simulink model "SimulinkSerial"  (R2019a)
settings: Solver=VariableStepAuto  StartTime=0.0  StopTime=inf  RelTol=1e-3
undefined symbols (not defined in the file): serial
libraries: instrumentlib x2
settings Model: Creator=JackyL  LastModifiedBy=Administrator
settings DataIOCC: ReturnWorkspaceOutputs=off
settings DebuggingCC: ArithmeticOperatorsInVariantConditions=warning

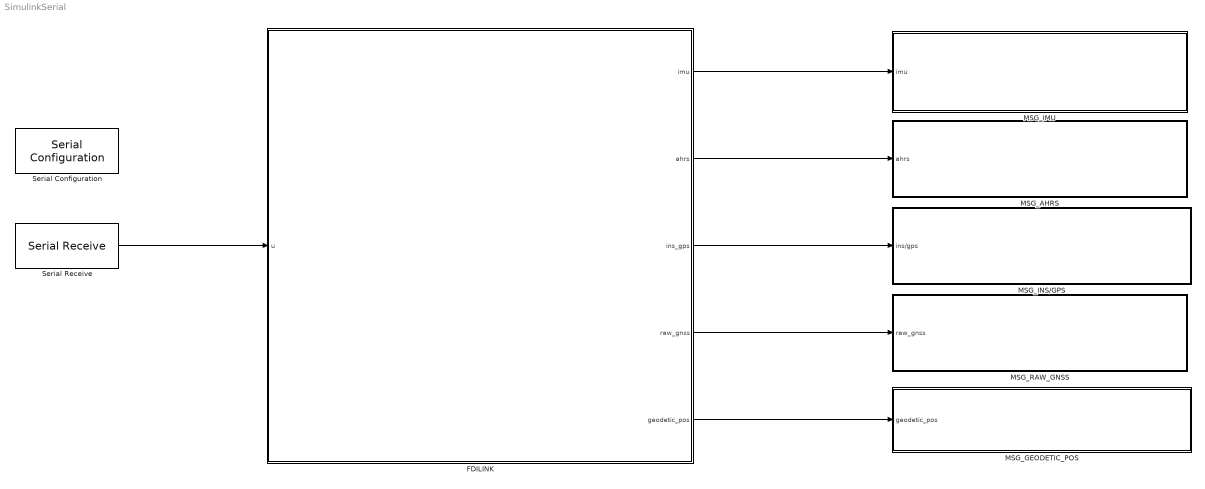
== system SimulinkSerial ==
  FDILINK : MATLAB Function  TreatAsAtomicUnit=on
  "MSG_AHRS " : Subsystem
  MSG_GEODETIC_POS : Subsystem
  "MSG_IMU " : Subsystem
  MSG_INS/GPS : Subsystem
  MSG_RAW_GNSS : Subsystem
  Serial Configuration : instrumentlib/Serial Configuration  Priority=-200000  ComPortMenu=<Please select a port...>  ComPort=COM2  ObjConstructor=serial('COM2');  BaudRate=921600  DataBits=8  Parity=none  StopBits=1  FlowControl=none  Timeout=10  ByteOrder=LittleEndian
  Serial Receive : instrumentlib/Serial Receive  ComPortMenu=COM2  ComPort=COM2  ObjConstructor=serial('COM2');  Terminator=<none>  DataSize="[1  200]"  DataType=uint8  EnableBlockingMode=on  ActionDataUnavailable=Output last received value  CustomValue=0  SampleTime=1
  wires:
  Serial Receive/1 -> FDILINK/1(u)
  FDILINK/1(imu) -> "MSG_IMU "/1("imu ")
  FDILINK/2(ahrs) -> "MSG_AHRS "/1("ahrs ")
  FDILINK/3(ins_gps) -> MSG_INS/GPS/1("ins/gps ")
  FDILINK/5(geodetic_pos) -> MSG_GEODETIC_POS/1("geodetic_pos ")
  FDILINK/4(raw_gnss) -> MSG_RAW_GNSS/1("raw_gnss ")

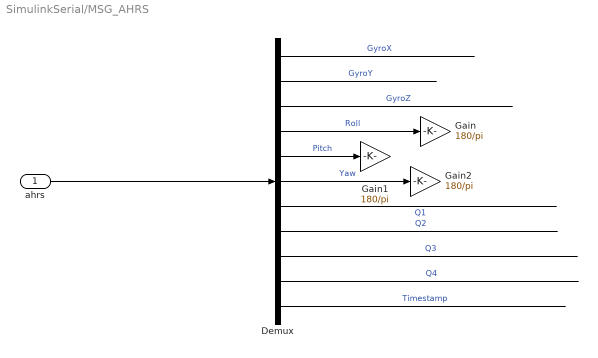
== system SimulinkSerial/MSG_AHRS  ==
  "ahrs " : Inport
  Demux : Demux  Outputs=11
  Gain : Gain  Gain=180/pi
  Gain1 : Gain  Gain=180/pi
  Gain2 : Gain  Gain=180/pi
  wires:
  "ahrs "/1 -> Demux/1
  Demux/1 -> ?  "GyroX"
  Demux/2 -> ?  "GyroY"
  Demux/3 -> ?  "GyroZ"
  Demux/5 -> Gain1/1  "Pitch"
  Demux/7 -> ?  "Q1"
  Demux/8 -> ?  "Q2"
  Demux/9 -> ?  "Q3"
  Demux/10 -> ?  "Q4"
  Demux/11 -> ?  "Timestamp"
  Demux/4 -> Gain/1  "Roll"
  Demux/6 -> Gain2/1  "Yaw"

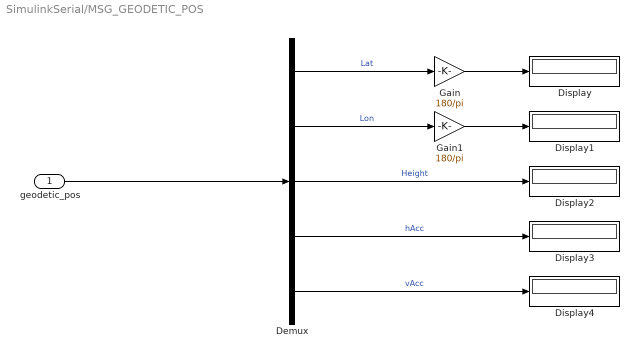
== system SimulinkSerial/MSG_GEODETIC_POS ==
  "geodetic_pos " : Inport
  Demux : Demux  Outputs=5
  Display{,1..4} (5 alike) : Display
  Gain : Gain  Gain=180/pi
  Gain1 : Gain  Gain=180/pi
  wires:
  "geodetic_pos "/1 -> Demux/1
  Demux/1 -> Gain/1  "Lat"
  Demux/3 -> Display2/1  "Height"
  Demux/4 -> Display3/1  "hAcc"
  Demux/2 -> Gain1/1  "Lon"
  Gain/1 -> Display/1
  Gain1/1 -> Display1/1
  Demux/5 -> Display4/1  "vAcc"

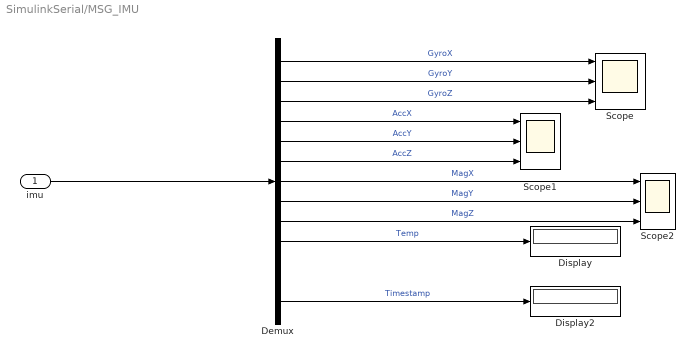
== system SimulinkSerial/MSG_IMU  ==
  "imu " : Inport
  Demux : Demux  Outputs=13
  Display : Display
  Display2 : Display
  Scope : Scope  NumInputPorts=3
  Scope1 : Scope  NumInputPorts=3
  Scope2 : Scope  NumInputPorts=3
  wires:
  "imu "/1 -> Demux/1
  Demux/2 -> Scope/2  "GyroY"
  Demux/10 -> Display/1  "Temp"
  Demux/8 -> Scope2/2  "MagY"
  Demux/5 -> Scope1/2  "AccY"
  Demux/7 -> Scope2/1  "MagX"
  Demux/6 -> Scope1/3  "AccZ"
  Demux/9 -> Scope2/3  "MagZ"
  Demux/3 -> Scope/3  "GyroZ"
  Demux/4 -> Scope1/1  "AccX"
  Demux/1 -> Scope/1  "GyroX"
  Demux/13 -> Display2/1  "Timestamp"

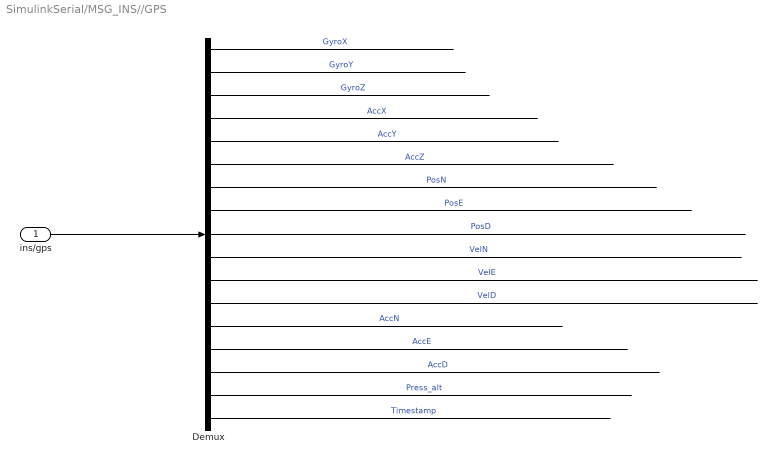
== system SimulinkSerial/MSG_INS//GPS ==
  "ins/gps " : Inport
  Demux : Demux  Outputs=17
  wires:
  "ins/gps "/1 -> Demux/1
  Demux/1 -> ?  "GyroX"
  Demux/2 -> ?  "GyroY"
  Demux/3 -> ?  "GyroZ"
  Demux/4 -> ?  "AccX"
  Demux/5 -> ?  "AccY"
  Demux/6 -> ?  "AccZ"
  Demux/7 -> ?  "PosN"
  Demux/8 -> ?  "PosE"
  Demux/9 -> ?  "PosD"
  Demux/10 -> ?  "VelN"
  Demux/11 -> ?  "VelE"
  Demux/12 -> ?  "VelD"
  Demux/13 -> ?  "AccN"
  Demux/14 -> ?  "AccE"
  Demux/15 -> ?  "AccD"
  Demux/16 -> ?  "Press_alt"
  Demux/17 -> ?  "Timestamp"

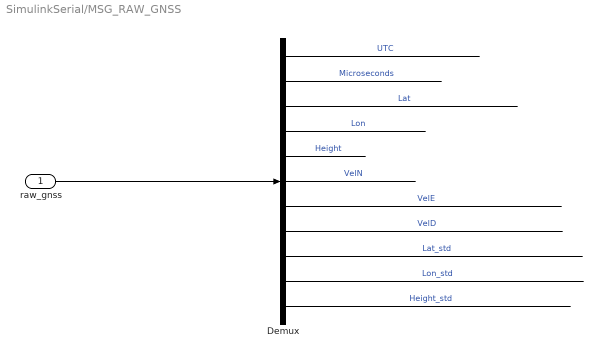
== system SimulinkSerial/MSG_RAW_GNSS ==
  "raw_gnss " : Inport
  Demux : Demux  Outputs=11
  wires:
  "raw_gnss "/1 -> Demux/1
  Demux/1 -> ?  "UTC"
  Demux/2 -> ?  "Microseconds"
  Demux/3 -> ?  "Lat"
  Demux/5 -> ?  "Height"
  Demux/7 -> ?  "VelE"
  Demux/8 -> ?  "VelD"
  Demux/9 -> ?  "Lat_std"
  Demux/10 -> ?  "Lon_std"
  Demux/11 -> ?  "Height_std"
  Demux/4 -> ?  "Lon"
  Demux/6 -> ?  "VelN"

== matlab function SimulinkSerial/FDILINK ==
  data: imu output; u input; ahrs output; ins_gps output; raw_gnss output; geodetic_pos output
function [imu,ahrs,ins_gps,raw_gnss,geodetic_pos] = fcn(u)
persistent FStatus;
persistent ReceiveDataLeft;
persistent ReceiveType;
persistent Buffer;
persistent BufferIndex;
persistent lastImu;
persistent lastAhrs;
persistent lastInsGps;
persistent lastRawGnss;
persistent lastGeodeticPos;
if isempty(FStatus)
	FStatus = 0;
	ReceiveDataLeft = uint8(0);
	BufferIndex = uint8(0);
	Buffer = uint8(zeros(1,256));
	ReceiveType = uint8(0);
	lastImu  = zeros(13,1);
    lastAhrs = zeros(11,1);
    lastInsGps = zeros(17,1);
    lastRawGnss = zeros(11,1);
    lastGeodeticPos = zeros(5,1);
end
%数据帧帧头FC
SerialBoot_STX_Flag = uint8(252);
%数据帧帧尾FD
SerialBoot_EDX_Flag = uint8(253);
for i = 1:length(u)
	value = u(i);
	switch (FStatus)
		case 0
			ReceiveDataLeft = uint8(0);
			if value == SerialBoot_STX_Flag
				FStatus = 1;
			end
		case 1
        %ReceiveType对应数据帧里的指令类别，比如IMU数据包为0x40，AHRS数据包为0x41，转化为十进制就是64和65；
			ReceiveType = value;
			FStatus = 2;
		case 2
        %ReceiveDataLeft对应数据帧里的暂未复制带Buffer里的数据长度（位），此时被赋予的值对应该数据包完整的数据长度；
			ReceiveDataLeft = value;
			BufferIndex = uint8(1);
			FStatus = 3;
		case 3
			FStatus = 4;
		case 4
			if ReceiveDataLeft == 0
				FStatus = 0;
			else
				FStatus = 5;
			end
		case 5
			FStatus = 6;
		case 6
			FStatus = 7;
		case 7
        %对应数据帧里的载荷，此时Buffer数据按顺序存储载荷里的数据直到全部复制完成
			Buffer(BufferIndex) = value;
			BufferIndex = BufferIndex + 1;
			ReceiveDataLeft = ReceiveDataLeft - 1;
			if ReceiveDataLeft == 0
				FStatus = 8;
			end
		case 8
			if (value == SerialBoot_EDX_Flag)
				switch(ReceiveType)
					case 64
						%% 解析MSG_IMU
						lastImu(1) = typecast(Buffer(1:4),'single');
						lastImu(2) = typecast(Buffer(5:8),'single');
						lastImu(3) = typecast(Buffer(9:12),'single');
						lastImu(4) = typecast(Buffer(13:16),'single');
						lastImu(5) = typecast(Buffer(17:20),'single');
						lastImu(6) = typecast(Buffer(21:24),'single');
						lastImu(7) = typecast(Buffer(25:28),'single');
						lastImu(8) = typecast(Buffer(29:32),'single');
						lastImu(9) = typecast(Buffer(33:36),'single');
						lastImu(10) = typecast(Buffer(37:40),'single');
						lastImu(11) = typecast(Buffer(41:44),'single');
                        lastImu(12) = typecast(Buffer(45:48),'single');
                        lastImu(13) = typecast(Buffer(49:56),'uint64');
					case 65
						%% 解析MSG_AHRS
						lastAhrs(1) = typecast(Buffer(1:4),'single');
						lastAhrs(2) = typecast(Buffer(5:8),'single');
						lastAhrs(3) = typecast(Buffer(9:12),'single');
						lastAhrs(4) = typecast(Buffer(13:16),'single');
						lastAhrs(5) = typecast(Buffer(17:20),'single');
						lastAhrs(6) = typecast(Buffer(21:24),'single');
						lastAhrs(7) = typecast(Buffer(25:28),'single');
						lastAhrs(8) = typecast(Buffer(29:32),'single');
						lastAhrs(9) = typecast(Buffer(33:36),'single');
						lastAhrs(10) = typecast(Buffer(37:40),'single');
                        lastAhrs(11) = typecast(Buffer(41:48),'uint64');
					case 66
						%% 解析MSG_INS/GPS
						lastInsGps(1) = typecast(Buffer(1:4),'single');
						lastInsGps(2) = typecast(Buffer(5:8),'single');
						lastInsGps(3) = typecast(Buffer(9:12),'single');
						lastInsGps(4) = typecast(Buffer(13:16),'single');
						lastInsGps(5) = typecast(Buffer(17:20),'single');
						lastInsGps(6) = typecast(Buffer(21:24),'single');
						lastInsGps(7) = typecast(Buffer(25:28),'single');
						lastInsGps(8) = typecast(Buffer(29:32),'single');
						lastInsGps(9) = typecast(Buffer(33:36),'single');
						lastInsGps(10) = typecast(Buffer(37:40),'single');
                        lastInsGps(11) = typecast(Buffer(41:44),'single');
                        lastInsGps(12) = typecast(Buffer(45:48),'single');
                        lastInsGps(13) = typecast(Buffer(49:52),'single');
                        lastInsGps(14) = typecast(Buffer(53:56),'single');
                        lastInsGps(15) = typecast(Buffer(57:60),'single');
                        lastInsGps(16) = typecast(Buffer(61:64),'single');
                        lastInsGps(17) = typecast(Buffer(65:72),'uint64');
					case 89
						%% 解析MSG_RAW_GNSS
						lastRawGnss(1) = typecast(Buffer(1:4),'uint32');
						lastRawGnss(2) = typecast(Buffer(5:8),'uint32');
						lastRawGnss(3) = typecast(Buffer(9:16),'double');
						lastRawGnss(4) = typecast(Buffer(17:24),'double');
						lastRawGnss(5) = typecast(Buffer(25:32),'double');
						lastRawGnss(6) = typecast(Buffer(33:36),'single');
						lastRawGnss(7) = typecast(Buffer(37:40),'single');
						lastRawGnss(8) = typecast(Buffer(41:44),'single');
						lastRawGnss(9) = typecast(Buffer(45:48),'single');
						lastRawGnss(10) = typecast(Buffer(49:52),'single');
                        lastRawGnss(11) = typecast(Buffer(53:56),'single');
					case 92
						%% 解析MSG_GEODETIC_POS
						lastGeodeticPos(1) = typecast(Buffer(1:8),'double');
						lastGeodeticPos(2) = typecast(Buffer(9:16),'double');
						lastGeodeticPos(3) = typecast(Buffer(17:24),'double');
						lastGeodeticPos(4) = typecast(Buffer(25:28),'single');
						lastGeodeticPos(5) = typecast(Buffer(29:32),'single');
                end	
			end
			FStatus = 0;
    end 
end

imu = lastImu;
ahrs = lastAhrs;
ins_gps = lastInsGps;
raw_gnss = lastRawGnss;
geodetic_pos = lastGeodeticPos;

end
